simulink model "rebuilt_model_comparison"  (R2013b)
settings: Solver=ode45  StartTime=0.0  StopTime=10.0  MaxStep=1e-4  RelTol=1e-6
values from neighbouring files (symbols this model uses):
  d = 0.5    [rebuilt__model_vars.mat]
  df = 0.2    [rebuilt__model_vars.mat]
  k = 5    [rebuilt__model_vars.mat]
  kf = 2    [rebuilt__model_vars.mat]
  m = 1    [rebuilt__model_vars.mat]
undefined symbols (not defined in the file or in its folder): d1, d2
settings Model: Creator=JNB  LastModifiedBy=JNB

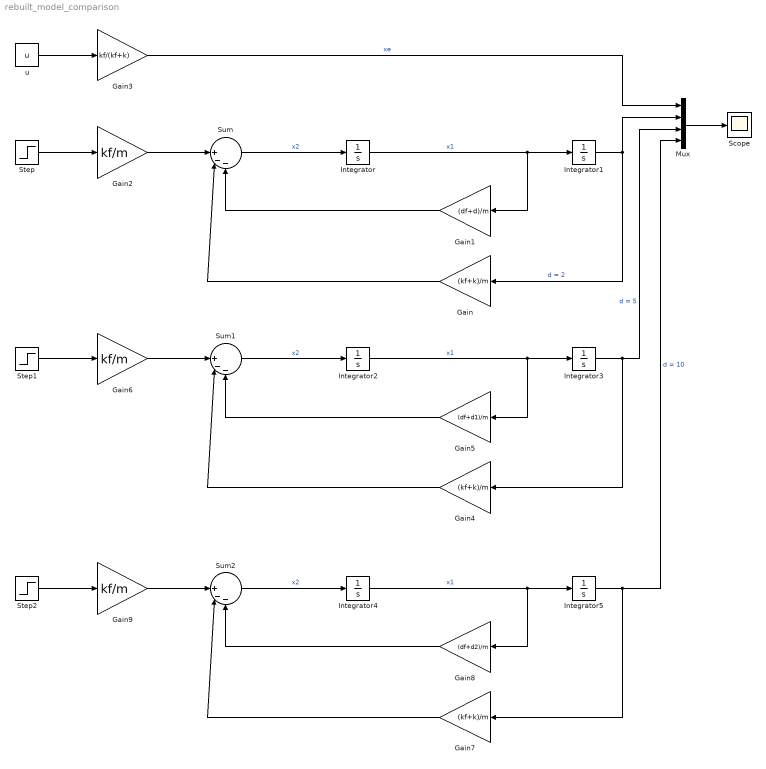
== system rebuilt_model_comparison ==
  Gain : Gain  Gain=(kf+k)/m
  Gain1 : Gain  Gain=(df+d)/m
  Gain2 : Gain  Gain=kf/m
  Gain3 : Gain  Gain=kf/(kf+k)
  Gain4 : Gain  Gain=(kf+k)/m
  Gain5 : Gain  Gain=(df+d1)/m
  Gain6 : Gain  Gain=kf/m
  Gain7 : Gain  Gain=(kf+k)/m
  Gain8 : Gain  Gain=(df+d2)/m
  Gain9 : Gain  Gain=kf/m
  Integrator{,1..5} (6 alike) : Integrator
  Mux : Mux
  Scope : Scope
      settings: ShowLegends=on
  Step : Step  SampleTime=0
  Step1 : Step  SampleTime=0
  Step2 : Step  SampleTime=0
  Sum : Sum  Inputs=||+--
  Sum1 : Sum  Inputs=||+--
  Sum2 : Sum  Inputs=||+--
  u : Constant  Value=u
  wires:
  Integrator/1 -> Gain1/1, Integrator1/1  "x1"
  Integrator1/1 -> Gain/1, Mux/2  "d = 2"
  Gain2/1 -> Sum/1
  Sum/1 -> Integrator/1  "x2"
  Gain1/1 -> Sum/3
  Gain/1 -> Sum/2
  Mux/1 -> Scope/1
  Step/1 -> Gain2/1
  u/1 -> Gain3/1
  Gain3/1 -> Mux/1  "xe"
  Integrator2/1 -> Gain5/1, Integrator3/1  "x1"
  Integrator3/1 -> Mux/3, Gain4/1  "d = 5"
  Gain6/1 -> Sum1/1
  Sum1/1 -> Integrator2/1  "x2"
  Gain5/1 -> Sum1/3
  Gain4/1 -> Sum1/2
  Step1/1 -> Gain6/1
  Integrator4/1 -> Gain8/1, Integrator5/1  "x1"
  Integrator5/1 -> Mux/4, Gain7/1  "d = 10"
  Gain9/1 -> Sum2/1
  Sum2/1 -> Integrator4/1  "x2"
  Gain8/1 -> Sum2/3
  Gain7/1 -> Sum2/2
  Step2/1 -> Gain9/1
